simulink model "valve_engine"  (R2023b)
settings: Solver=VariableStepAuto  StartTime=0.0  StopTime=10.0  RelTol=1e-3
values from neighbouring files (symbols this model uses):
  I = 0    [engine_model_param.m]    (also in parameters.m = 0.0001796625)
  K_t = 0.218    [engine_model_param.m]    (also in parameters.m)
  nominal_current = 3.5    [engine_model_param.m]    (also in parameters.m)
  nominal_torque = 0.75    [engine_model_param.m]    (also in parameters.m)
  nominal_voltage = 48    [engine_model_param.m]    (also in parameters.m)
  pairs = 20    [engine_model_param.m]    (also in parameters.m)
  rotation_speed = 1820 / 60    (= 30.3333333333)    [engine_model_param.m]    (also in parameters.m)
settings Model: Creator=kirill  LastModifiedBy=kirill

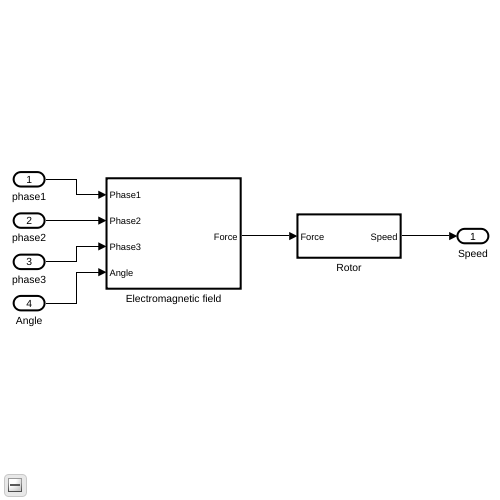
[thumbnail: Simulink's stored preview of the top-level diagram]
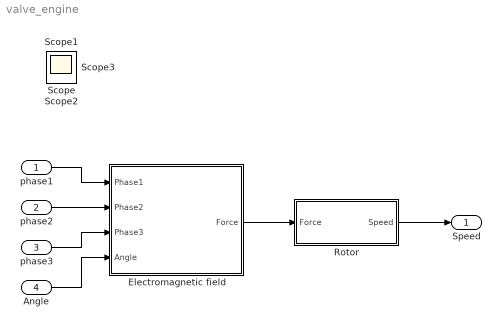
== system valve_engine ==
  phase1 : Inport
  phase2 : Inport  Port=2
  phase3 : Inport  Port=3
  Angle : Inport  Port=4
  Electromagnetic field : Subsystem
  Rotor : Subsystem
  Speed : Outport
  Scope{,1..3} (4 alike) : Scope
  wires:
  phase1/1 -> Electromagnetic field/1(Phase1)
  phase2/1 -> Electromagnetic field/2(Phase2)
  phase3/1 -> Electromagnetic field/3(Phase3)
  Rotor/1(Speed) -> Speed/1
  Electromagnetic field/1(Force) -> Rotor/1(Force)
  Angle/1 -> Electromagnetic field/4(Angle)

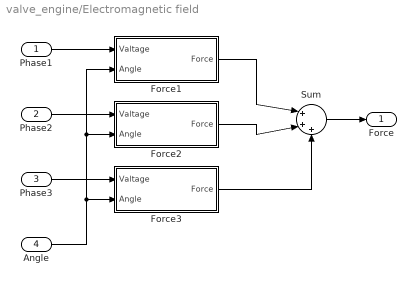
== system valve_engine/Electromagnetic field ==
  Phase1 : Inport
  Phase2 : Inport  Port=2
  Phase3 : Inport  Port=3
  Angle : Inport  Port=4
  Force1 : Subsystem
  Force2 : Subsystem
  Force3 : Subsystem
  Sum : Sum  Inputs=|+++
  Force : Outport
  wires:
  Phase1/1 -> Force1/1(Valtage)
  Angle/1 -> Force3/2(Angle), Force2/2(Angle), Force1/2(Angle)
  Phase3/1 -> Force3/1(Valtage)
  Force1/1(Force) -> Sum/1
  Force2/1(Force) -> Sum/2
  Force3/1(Force) -> Sum/3
  Sum/1 -> Force/1
  Phase2/1 -> Force2/1(Valtage)

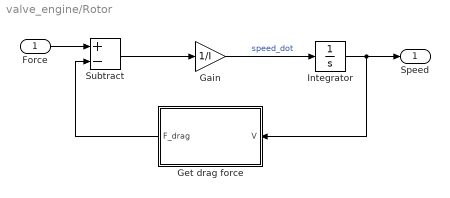
== system valve_engine/Rotor ==
  Force : Inport
  Gain : Gain  Gain=1/I
  Get drag force : MATLAB Function  TreatAsAtomicUnit=on
  Integrator : Integrator
  Subtract : Sum  Inputs=+-
  Speed : Outport
  wires:
  Force/1 -> Subtract/1
  Subtract/1 -> Gain/1
  Gain/1 -> Integrator/1  "speed_dot"
  Integrator/1 -> Get drag force/1(V), Speed/1
  Get drag force/1(F_drag) -> Subtract/2

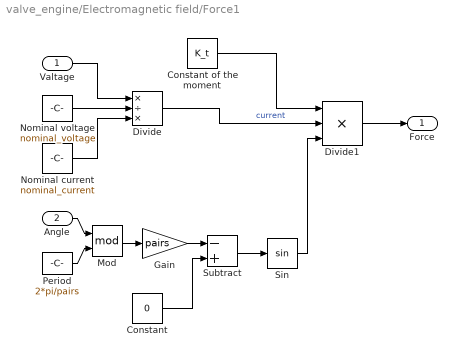
== system valve_engine/Electromagnetic field/Force1 ==
  Valtage : Inport
  Angle : Inport  Port=2
  Constant : Constant  Value=0
  Divide : Product  Inputs=*/*  RndMeth=Zero  SaturateOnIntegerOverflow=on
  Divide1 : Product  Inputs=***
  Gain : Gain  Gain=pairs
  Mod : Math  Operator=mod
  Nominal current : Constant  Value=nominal_current
  Nominal voltage : Constant  Value=nominal_voltage
  Period : Constant  Value=2*pi/pairs
  Sin : Trigonometry
  Subtract : Sum  Inputs=-+
  Сonstant of the moment : Constant  Value=K_t
  Force : Outport
  wires:
  Сonstant of the moment/1 -> Divide1/1
  Divide/1 -> Divide1/2  "current"
  Divide1/1 -> Force/1
  Sin/1 -> Divide1/3
  Valtage/1 -> Divide/1
  Nominal voltage/1 -> Divide/2
  Nominal current/1 -> Divide/3
  Angle/1 -> Mod/1
  Period/1 -> Mod/2
  Mod/1 -> Gain/1
  Gain/1 -> Subtract/1
  Constant/1 -> Subtract/2
  Subtract/1 -> Sin/1

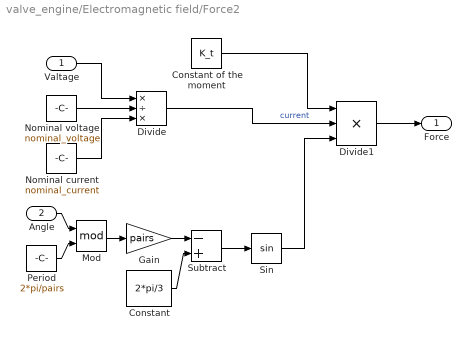
== system valve_engine/Electromagnetic field/Force2 ==
  Valtage : Inport
  Angle : Inport  Port=2
  Constant : Constant  Value=2*pi/3
  Divide : Product  Inputs=*/*  RndMeth=Zero  SaturateOnIntegerOverflow=on
  Divide1 : Product  Inputs=***
  Gain : Gain  Gain=pairs
  Mod : Math  Operator=mod
  Nominal current : Constant  Value=nominal_current
  Nominal voltage : Constant  Value=nominal_voltage
  Period : Constant  Value=2*pi/pairs
  Sin : Trigonometry
  Subtract : Sum  Inputs=-+
  Сonstant of the moment : Constant  Value=K_t
  Force : Outport
  wires:
  Nominal current/1 -> Divide/3
  Divide/1 -> Divide1/2  "current"
  Nominal voltage/1 -> Divide/2
  Сonstant of the moment/1 -> Divide1/1
  Divide1/1 -> Force/1
  Valtage/1 -> Divide/1
  Sin/1 -> Divide1/3
  Period/1 -> Mod/2
  Gain/1 -> Subtract/1
  Mod/1 -> Gain/1
  Angle/1 -> Mod/1
  Constant/1 -> Subtract/2
  Subtract/1 -> Sin/1

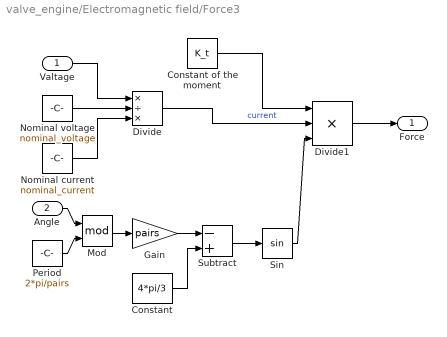
== system valve_engine/Electromagnetic field/Force3 ==
  Valtage : Inport
  Angle : Inport  Port=2
  Constant : Constant  Value=4*pi/3
  Divide : Product  Inputs=*/*  RndMeth=Zero  SaturateOnIntegerOverflow=on
  Divide1 : Product  Inputs=***
  Gain : Gain  Gain=pairs
  Mod : Math  Operator=mod
  Nominal current : Constant  Value=nominal_current
  Nominal voltage : Constant  Value=nominal_voltage
  Period : Constant  Value=2*pi/pairs
  Sin : Trigonometry
  Subtract : Sum  Inputs=-+
  Сonstant of the moment : Constant  Value=K_t
  Force : Outport
  wires:
  Nominal current/1 -> Divide/3
  Subtract/1 -> Sin/1
  Divide/1 -> Divide1/2  "current"
  Nominal voltage/1 -> Divide/2
  Сonstant of the moment/1 -> Divide1/1
  Divide1/1 -> Force/1
  Valtage/1 -> Divide/1
  Sin/1 -> Divide1/3
  Period/1 -> Mod/2
  Gain/1 -> Subtract/1
  Mod/1 -> Gain/1
  Angle/1 -> Mod/1
  Constant/1 -> Subtract/2

== matlab function valve_engine/Rotor/Get drag force ==
  data: V input; F_drag output; nominal_torque parameter; rotation_speed parameter
function F_drag = get_drag_force(V, nominal_torque, rotation_speed)
k_drag = nominal_torque / (rotation_speed ^ 2);
F_drag = k_drag * V * abs(V);
